simulink library "cmlib"  (Simulink 6.0)
undefined symbols (not defined in the file or in its folder): get_linearcon_param, linearcon
settings Model: Creator=Zhan  LastModifiedBy=Zhan

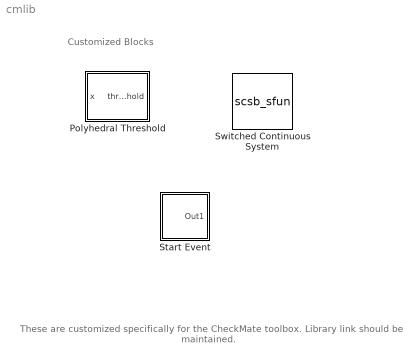
== system cmlib ==
  note: Customized Blocks
  note: These are customized specifically for the CheckMate toolbox.
      | Library link should be maintained.
  Polyhedral Threshold : Subsystem  mask(PolyhedralThreshold){polyhedron=floor}
      mask prompts: polyhedron "Polyhedron (@linearcon from work space)"
      mask help: This block represents a closed polyhedral region of the form C*x <= d. See the CheckMate documentation in the "/CheckMate/doc/" directory for a complete description of this block.
      mask Display: plot(poly_icon(1),poly_icon(2)); disp('C*x <= d')
  Start Event : Subsystem  TreatAsAtomicUnit=on  mask(Start event){steptime=1, initval=0, finival=1, sampletime=0, interpret=on, enable=on}
      mask prompts: steptime "Step time:"; initval "Initial value:"; finival "Final value:"; sampletime "Sample time:"; interpret "Interpret vector parameter as 1D"; enable "Enable zero crossing detection"
      mask help: Output a step.
      mask Help: Outputs a step from false to true.
      mask Display: plot([0 1 1 2],[0 0 0.5 0.5])
  Switched Continuous System : S-Function  AncestorBlock=cmlib/Switched Continuous System  FunctionName=scsb_sfun  Parameters=nx,nup,nz,nu,x0,swfunc,p0,use_reset,use_param,use_sd,get_linearcon_param(AR,'CI'),get_linearcon_param(AR,'dI')  EnableBusSupport=off  mask(SwitchedContinuousSystem){nx=1, use_sd=off, nup=[], nz=[], use_reset=on, nu=1, x0=1, swfunc=, ICS=linearcon, AR=linearcon, use_param=off, p0=[], PaCs=[], np=}
      mask prompts: nx "Number of Continuous States"; use_sd "Perform Sampled-Data Difference Equation Analysis (beta version)"; nup "Number of Controller Outputs"; nz "Number of Discrete-Time Controller States"; use_reset "Show State Reset Port"; nu "Number of Integer Inputs from Stateflow Blocks"; x0 "Initial Conditions"; swfunc "Switching Function m-file"; ICS "Initial Continuous Set (@linearcon cell array from workspace)"; AR "Analysis Region (@linearcon from work space)"; use_param "Use Parameter Constraints"; p0 "Default Parameter"; PaCs "Parameter Constraints (@ linearcon from workspace)"; np "Old Parameter"
      mask help: This block represents a switched continuous dynamic system. The switching function is m-file function f(x,u) that outputs the continuous derivative xdot given continuous variable x and discrete (integer) input u. Initial continuous set and analysis region parameters are used for PIHA conversion purpose only. They do not affect the simulation result. They must be @linearcon objects imported from the main workspace in the MATLAB command window.
      mask init:
      | scsb_mask_handler(gcb)
      mask Display: plot(scsb_icon(1),scsb_icon(2))

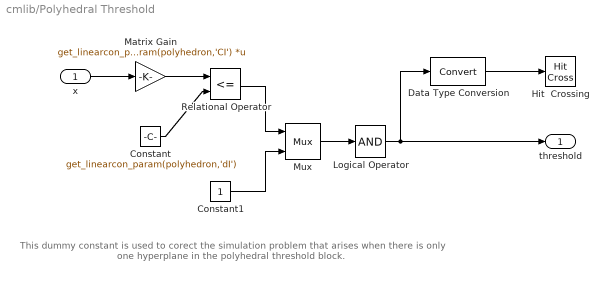
== system cmlib/Polyhedral Threshold ==
  note: This dummy constant is used to corect
      | the simulation problem that arises when
      | there is only one hyperplane in the
      | polyhedral threshold block.
  x : Inport  OutDataType=sfix(16)  OutScaling=2^0
  Constant : Constant  Value=get_linearcon_param(polyhedron,'dI')  OutDataType=sfix(16)  OutScaling=2^0
  Constant1 : Constant  OutDataTypeMode=boolean  OutDataType=sfix(16)  OutScaling=2^0
  Data Type Conversion : DataTypeConversion  OutDataTypeMode=double  SaturateOnIntegerOverflow=on  RndMeth=Zero
  Hit  Crossing : HitCross  HitCrossingOffset=0.5  ShowOutputPort=off
  Logical Operator : Logic  Inputs=1
  Matrix Gain : Gain  Gain=get_linearcon_param(polyhedron,'CI')  Multiplication=Matrix(K*u)  ParameterDataType=sfix(16)  ParameterScaling=2^0  OutDataType=sfix(16)  OutScaling=2^0  SaturateOnIntegerOverflow=on
  Mux : Mux  Inputs=2
  Relational Operator : RelationalOperator  Operator=<=  LogicOutDataTypeMode=boolean  InputSameDT=on
  threshold : Outport  InitialOutput=0
  wires:
  Constant/1 -> Relational Operator/2
  Matrix Gain/1 -> Relational Operator/1
  x/1 -> Matrix Gain/1
  Constant1/1 -> Mux/2
  Relational Operator/1 -> Mux/1
  Mux/1 -> Logical Operator/1
  Logical Operator/1 -> Data Type Conversion/1, threshold/1
  Data Type Conversion/1 -> Hit  Crossing/1

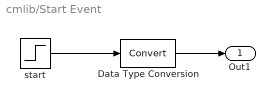
== system cmlib/Start Event ==
  Data Type Conversion : DataTypeConversion  OutDataTypeMode=boolean  SaturateOnIntegerOverflow=on  RndMeth=Zero
  start : Step  Time=steptime  Before=initval  After=finival  SampleTime=sampletime
  Out1 : Outport
  wires:
  Data Type Conversion/1 -> Out1/1
  start/1 -> Data Type Conversion/1
